simulink model "PWMGenerator"  (R2014b)
settings: Solver=ode45  StartTime=0.0  StopTime=2000  RelTol=1e-3
libraries: hdlsllib x15, simulink x5
settings Model: Creator=mchugh.ch  LastModifiedBy=sylvanus.a
settings OptimizationCC: UseDivisionForNetSlopeComputation=off  SimCompilerOptimization=off
settings DebuggingCC: FrameProcessingCompatibilityMsg=error
settings RTWCC: RTWCompilerOptimization=off
settings ConfigComp: CovMetricSettings=dw  CovHtmlReporting=on  CovSaveCumulativeToWorkspaceVar=on  CovSaveSingleToWorkspaceVar=on  CovModelRefEnable=Off  CovExternalEMLEnable=off  CovSFcnEnable=off

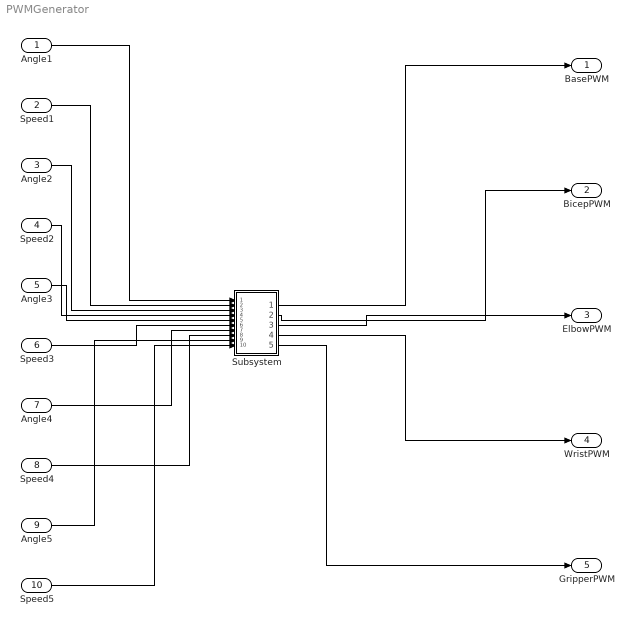
== system PWMGenerator ==
  Angle1 : Inport
  Speed1 : Inport  Port=2
  Angle2 : Inport  Port=3
  Speed2 : Inport  Port=4
  Angle3 : Inport  Port=5
  Speed3 : Inport  Port=6
  Angle4 : Inport  Port=7
  Speed4 : Inport  Port=8
  Angle5 : Inport  Port=9
  Speed5 : Inport  Port=10
  Subsystem : Subsystem  TreatAsAtomicUnit=on
  BasePWM : Outport  SampleTime=1
  BicepPWM : Outport  Port=2  SampleTime=1
  ElbowPWM : Outport  Port=3  SampleTime=1
  WristPWM : Outport  Port=4  SampleTime=1
  GripperPWM : Outport  Port=5  SampleTime=1
  wires:
  Angle1/1 -> Subsystem/1(Angle1)
  Speed1/1 -> Subsystem/2(Speed1)
  Angle2/1 -> Subsystem/3(Angle2)
  Speed2/1 -> Subsystem/4(Speed2)
  Angle3/1 -> Subsystem/5(Angle3)
  Speed3/1 -> Subsystem/6(Speed3)
  Angle4/1 -> Subsystem/7(Angle4)
  Speed4/1 -> Subsystem/8(Speed4)
  Angle5/1 -> Subsystem/9(Angle5)
  Speed5/1 -> Subsystem/10(Speed5)
  Subsystem/1(BasePWM) -> BasePWM/1
  Subsystem/2(BicepPWM) -> BicepPWM/1
  Subsystem/3(ElbowPWM) -> ElbowPWM/1
  Subsystem/4(WristPWM) -> WristPWM/1
  Subsystem/5(GripperPWM) -> GripperPWM/1

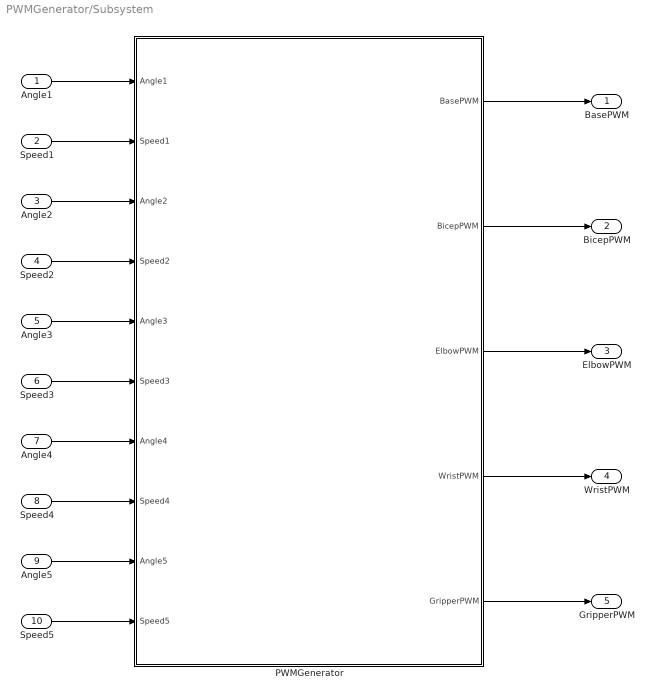
== system PWMGenerator/Subsystem ==
  Angle1 : Inport
  Speed1 : Inport  Port=2
  Angle2 : Inport  Port=3
  Speed2 : Inport  Port=4
  Angle3 : Inport  Port=5
  Speed3 : Inport  Port=6
  Angle4 : Inport  Port=7
  Speed4 : Inport  Port=8
  Angle5 : Inport  Port=9
  Speed5 : Inport  Port=10
  PWMGenerator : Subsystem
  BasePWM : Outport  SampleTime=1
  BicepPWM : Outport  Port=2  SampleTime=1
  ElbowPWM : Outport  Port=3  SampleTime=1
  WristPWM : Outport  Port=4  SampleTime=1
  GripperPWM : Outport  Port=5  SampleTime=1
  wires:
  Speed5/1 -> PWMGenerator/10(Speed5)
  PWMGenerator/5(GripperPWM) -> GripperPWM/1
  PWMGenerator/4(WristPWM) -> WristPWM/1
  PWMGenerator/2(BicepPWM) -> BicepPWM/1
  PWMGenerator/1(BasePWM) -> BasePWM/1
  PWMGenerator/3(ElbowPWM) -> ElbowPWM/1
  Speed3/1 -> PWMGenerator/6(Speed3)
  Angle3/1 -> PWMGenerator/5(Angle3)
  Angle2/1 -> PWMGenerator/3(Angle2)
  Speed1/1 -> PWMGenerator/2(Speed1)
  Angle4/1 -> PWMGenerator/7(Angle4)
  Speed4/1 -> PWMGenerator/8(Speed4)
  Angle5/1 -> PWMGenerator/9(Angle5)
  Angle1/1 -> PWMGenerator/1(Angle1)
  Speed2/1 -> PWMGenerator/4(Speed2)

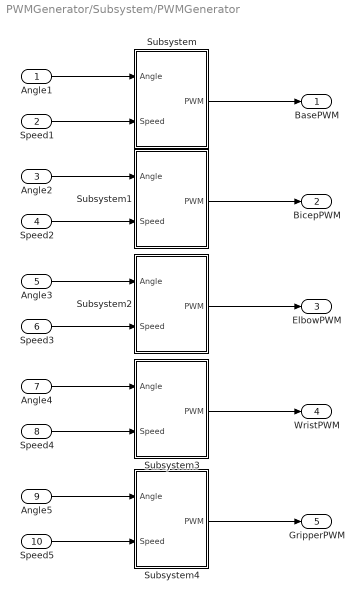
== system PWMGenerator/Subsystem/PWMGenerator ==
  Angle1 : Inport
  Speed1 : Inport  Port=2
  Angle2 : Inport  Port=3
  Speed2 : Inport  Port=4
  Angle3 : Inport  Port=5
  Speed3 : Inport  Port=6
  Angle4 : Inport  Port=7
  Speed4 : Inport  Port=8
  Angle5 : Inport  Port=9
  Speed5 : Inport  Port=10
  Subsystem : Subsystem  TreatAsAtomicUnit=on
  Subsystem1 : Subsystem  TreatAsAtomicUnit=on
  Subsystem2 : Subsystem  TreatAsAtomicUnit=on
  Subsystem3 : Subsystem  TreatAsAtomicUnit=on
  Subsystem4 : Subsystem  TreatAsAtomicUnit=on
  BasePWM : Outport  SampleTime=1
  BicepPWM : Outport  Port=2  SampleTime=1
  ElbowPWM : Outport  Port=3  SampleTime=1
  WristPWM : Outport  Port=4  SampleTime=1
  GripperPWM : Outport  Port=5  SampleTime=1
  wires:
  Speed1/1 -> Subsystem/2(Speed)
  Speed5/1 -> Subsystem4/2(Speed)
  Angle5/1 -> Subsystem4/1(Angle)
  Subsystem4/1(PWM) -> GripperPWM/1
  Angle1/1 -> Subsystem/1(Angle)
  Angle3/1 -> Subsystem2/1(Angle)
  Subsystem2/1(PWM) -> ElbowPWM/1
  Speed3/1 -> Subsystem2/2(Speed)
  Speed2/1 -> Subsystem1/2(Speed)
  Subsystem1/1(PWM) -> BicepPWM/1
  Angle2/1 -> Subsystem1/1(Angle)
  Subsystem3/1(PWM) -> WristPWM/1
  Angle4/1 -> Subsystem3/1(Angle)
  Speed4/1 -> Subsystem3/2(Speed)
  Subsystem/1(PWM) -> BasePWM/1

== system PWMGenerator/Subsystem/PWMGenerator/Subsystem ==
  Angle : Inport  OutDataTypeStr=uint32  SampleTime=1
  Speed : Inport  Port=2  OutDataTypeStr=uint32  SampleTime=1
  AngleSpeedToPWM : Subsystem
  Scope : Scope
  PWM : Outport  SampleTime=1
  wires:
  Speed/1 -> AngleSpeedToPWM/2(Speed)
  Angle/1 -> AngleSpeedToPWM/1(Angle)
  AngleSpeedToPWM/1(PWM) -> PWM/1, Scope/1

== system PWMGenerator/Subsystem/PWMGenerator/Subsystem1 ==
  Angle : Inport  OutDataTypeStr=uint32  SampleTime=1
  Speed : Inport  Port=2  OutDataTypeStr=uint32  SampleTime=1
  AngleSpeedToPWM : Subsystem
  Scope : Scope
  PWM : Outport  SampleTime=1
  wires:
  Speed/1 -> AngleSpeedToPWM/2(Speed)
  Angle/1 -> AngleSpeedToPWM/1(Angle)
  AngleSpeedToPWM/1(PWM) -> PWM/1, Scope/1

== system PWMGenerator/Subsystem/PWMGenerator/Subsystem2 ==
  Angle : Inport  OutDataTypeStr=uint32  SampleTime=1
  Speed : Inport  Port=2  OutDataTypeStr=uint32  SampleTime=1
  AngleSpeedToPWM : Subsystem
  Scope : Scope
  PWM : Outport  SampleTime=1
  wires:
  Speed/1 -> AngleSpeedToPWM/2(Speed)
  Angle/1 -> AngleSpeedToPWM/1(Angle)
  AngleSpeedToPWM/1(PWM) -> PWM/1, Scope/1

== system PWMGenerator/Subsystem/PWMGenerator/Subsystem3 ==
  Angle : Inport  OutDataTypeStr=uint32  SampleTime=1
  Speed : Inport  Port=2  OutDataTypeStr=uint32  SampleTime=1
  AngleSpeedToPWM : Subsystem
  Scope : Scope
  PWM : Outport  SampleTime=1
  wires:
  Speed/1 -> AngleSpeedToPWM/2(Speed)
  Angle/1 -> AngleSpeedToPWM/1(Angle)
  AngleSpeedToPWM/1(PWM) -> PWM/1, Scope/1

== system PWMGenerator/Subsystem/PWMGenerator/Subsystem4 ==
  Angle : Inport  OutDataTypeStr=uint32  SampleTime=1
  Speed : Inport  Port=2  OutDataTypeStr=uint32  SampleTime=1
  AngleSpeedToPWM : Subsystem
  Scope : Scope
  PWM : Outport  SampleTime=1
  wires:
  Speed/1 -> AngleSpeedToPWM/2(Speed)
  Angle/1 -> AngleSpeedToPWM/1(Angle)
  AngleSpeedToPWM/1(PWM) -> PWM/1, Scope/1

== system PWMGenerator/Subsystem/PWMGenerator/Subsystem/AngleSpeedToPWM ==
  Angle : Inport  OutDataTypeStr=uint32  SampleTime=1
  Speed : Inport  Port=2  OutDataTypeStr=uint32  SampleTime=1
  Subsystem : Subsystem
  PWM : Outport  SampleTime=1
  wires:
  Angle/1 -> Subsystem/1(Angle)
  Speed/1 -> Subsystem/2(Speed)
  Subsystem/1(PWM) -> PWM/1

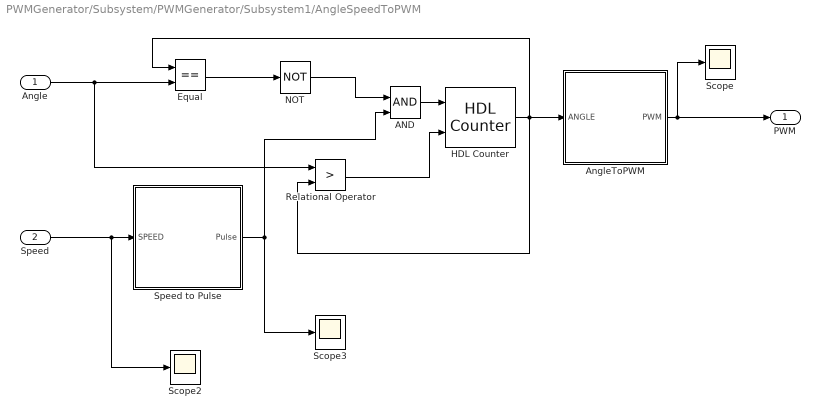
== system PWMGenerator/Subsystem/PWMGenerator/Subsystem1/AngleSpeedToPWM ==
  Angle : Inport  OutDataTypeStr=uint32  SampleTime=1
  Speed : Inport  Port=2  OutDataTypeStr=uint32  SampleTime=1
  AND : Logic  IconShape=distinctive  AllPortsSameDT=off  OutDataTypeStr=boolean
  AngleToPWM : Subsystem
  Equal : RelationalOperator  Operator===  OutDataTypeStr=boolean  SampleTime=1
  HDL Counter : hdlsllib/HDL Operations/HDL Counter  CountType=Count limited  CountInit=90  CountStep=1  CountMax=180  CountFromType=Specify  CountFrom=0  CountResetPort=off  CountLoadPort=off  CountEnbPort=on  CountDirPort=on  CountDataType=Unsigned  CountWordLen=32  CountFracLen=0  CountSampTime=1
  NOT : Logic  Operator=NOT  IconShape=distinctive  AllPortsSameDT=off  OutDataTypeStr=boolean
  Relational Operator : RelationalOperator  Operator=>  OutDataTypeStr=boolean
  Scope : Scope
      settings: SaveName=ScopeData5
  Scope2 : Scope
      settings: SaveName=ScopeData6
  Scope3 : Scope
      settings: SaveName=ScopeData7
  Speed to Pulse : Subsystem
  PWM : Outport  SampleTime=1
  wires:
  Equal/1 -> NOT/1
  HDL Counter/1 -> Relational Operator/2, Equal/1, AngleToPWM/1(ANGLE)
  AND/1 -> HDL Counter/1
  Speed/1 -> Scope2/1, Speed to Pulse/1(SPEED)
  Relational Operator/1 -> HDL Counter/2
  Speed to Pulse/1(Pulse) -> Scope3/1, AND/2
  NOT/1 -> AND/1
  AngleToPWM/1(PWM) -> PWM/1, Scope/1
  Angle/1 -> Equal/2, Relational Operator/1

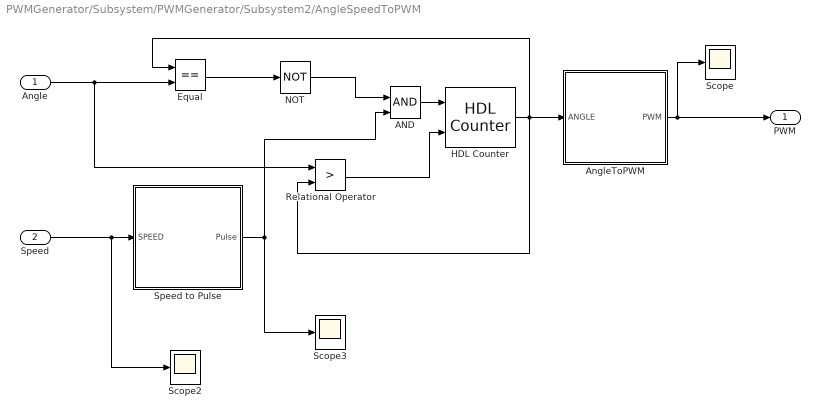
== system PWMGenerator/Subsystem/PWMGenerator/Subsystem2/AngleSpeedToPWM ==
  Angle : Inport  OutDataTypeStr=uint32  SampleTime=1
  Speed : Inport  Port=2  OutDataTypeStr=uint32  SampleTime=1
  AND : Logic  IconShape=distinctive  AllPortsSameDT=off  OutDataTypeStr=boolean
  AngleToPWM : Subsystem
  Equal : RelationalOperator  Operator===  OutDataTypeStr=boolean  SampleTime=1
  HDL Counter : hdlsllib/HDL Operations/HDL Counter  CountType=Count limited  CountInit=90  CountStep=1  CountMax=180  CountFromType=Specify  CountFrom=0  CountResetPort=off  CountLoadPort=off  CountEnbPort=on  CountDirPort=on  CountDataType=Unsigned  CountWordLen=32  CountFracLen=0  CountSampTime=1
  NOT : Logic  Operator=NOT  IconShape=distinctive  AllPortsSameDT=off  OutDataTypeStr=boolean
  Relational Operator : RelationalOperator  Operator=>  OutDataTypeStr=boolean
  Scope : Scope
      settings: SaveName=ScopeData5
  Scope2 : Scope
      settings: SaveName=ScopeData6
  Scope3 : Scope
      settings: SaveName=ScopeData7
  Speed to Pulse : Subsystem
  PWM : Outport  SampleTime=1
  wires:
  Equal/1 -> NOT/1
  HDL Counter/1 -> Relational Operator/2, Equal/1, AngleToPWM/1(ANGLE)
  AND/1 -> HDL Counter/1
  Speed/1 -> Scope2/1, Speed to Pulse/1(SPEED)
  Relational Operator/1 -> HDL Counter/2
  Speed to Pulse/1(Pulse) -> Scope3/1, AND/2
  NOT/1 -> AND/1
  AngleToPWM/1(PWM) -> PWM/1, Scope/1
  Angle/1 -> Equal/2, Relational Operator/1

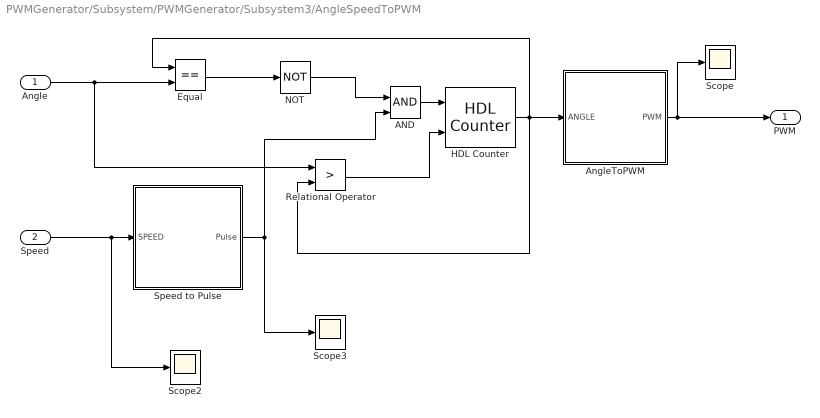
== system PWMGenerator/Subsystem/PWMGenerator/Subsystem3/AngleSpeedToPWM ==
  Angle : Inport  OutDataTypeStr=uint32  SampleTime=1
  Speed : Inport  Port=2  OutDataTypeStr=uint32  SampleTime=1
  AND : Logic  IconShape=distinctive  AllPortsSameDT=off  OutDataTypeStr=boolean
  AngleToPWM : Subsystem
  Equal : RelationalOperator  Operator===  OutDataTypeStr=boolean  SampleTime=1
  HDL Counter : hdlsllib/HDL Operations/HDL Counter  CountType=Count limited  CountInit=90  CountStep=1  CountMax=180  CountFromType=Specify  CountFrom=0  CountResetPort=off  CountLoadPort=off  CountEnbPort=on  CountDirPort=on  CountDataType=Unsigned  CountWordLen=32  CountFracLen=0  CountSampTime=1
  NOT : Logic  Operator=NOT  IconShape=distinctive  AllPortsSameDT=off  OutDataTypeStr=boolean
  Relational Operator : RelationalOperator  Operator=>  OutDataTypeStr=boolean
  Scope : Scope
      settings: SaveName=ScopeData5
  Scope2 : Scope
      settings: SaveName=ScopeData6
  Scope3 : Scope
      settings: SaveName=ScopeData7
  Speed to Pulse : Subsystem
  PWM : Outport  SampleTime=1
  wires:
  Equal/1 -> NOT/1
  HDL Counter/1 -> Relational Operator/2, Equal/1, AngleToPWM/1(ANGLE)
  AND/1 -> HDL Counter/1
  Speed/1 -> Scope2/1, Speed to Pulse/1(SPEED)
  Relational Operator/1 -> HDL Counter/2
  Speed to Pulse/1(Pulse) -> Scope3/1, AND/2
  NOT/1 -> AND/1
  AngleToPWM/1(PWM) -> PWM/1, Scope/1
  Angle/1 -> Equal/2, Relational Operator/1

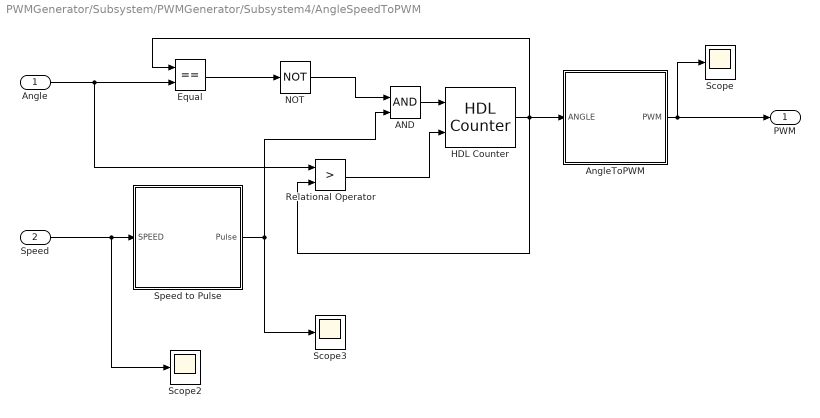
== system PWMGenerator/Subsystem/PWMGenerator/Subsystem4/AngleSpeedToPWM ==
  Angle : Inport  OutDataTypeStr=uint32  SampleTime=1
  Speed : Inport  Port=2  OutDataTypeStr=uint32  SampleTime=1
  AND : Logic  IconShape=distinctive  AllPortsSameDT=off  OutDataTypeStr=boolean
  AngleToPWM : Subsystem
  Equal : RelationalOperator  Operator===  OutDataTypeStr=boolean  SampleTime=1
  HDL Counter : hdlsllib/HDL Operations/HDL Counter  CountType=Count limited  CountInit=90  CountStep=1  CountMax=180  CountFromType=Specify  CountFrom=0  CountResetPort=off  CountLoadPort=off  CountEnbPort=on  CountDirPort=on  CountDataType=Unsigned  CountWordLen=32  CountFracLen=0  CountSampTime=1
  NOT : Logic  Operator=NOT  IconShape=distinctive  AllPortsSameDT=off  OutDataTypeStr=boolean
  Relational Operator : RelationalOperator  Operator=>  OutDataTypeStr=boolean
  Scope : Scope
      settings: SaveName=ScopeData5
  Scope2 : Scope
      settings: SaveName=ScopeData6
  Scope3 : Scope
      settings: SaveName=ScopeData7
  Speed to Pulse : Subsystem
  PWM : Outport  SampleTime=1
  wires:
  Equal/1 -> NOT/1
  HDL Counter/1 -> Relational Operator/2, Equal/1, AngleToPWM/1(ANGLE)
  AND/1 -> HDL Counter/1
  Speed/1 -> Scope2/1, Speed to Pulse/1(SPEED)
  Relational Operator/1 -> HDL Counter/2
  Speed to Pulse/1(Pulse) -> Scope3/1, AND/2
  NOT/1 -> AND/1
  AngleToPWM/1(PWM) -> PWM/1, Scope/1
  Angle/1 -> Equal/2, Relational Operator/1

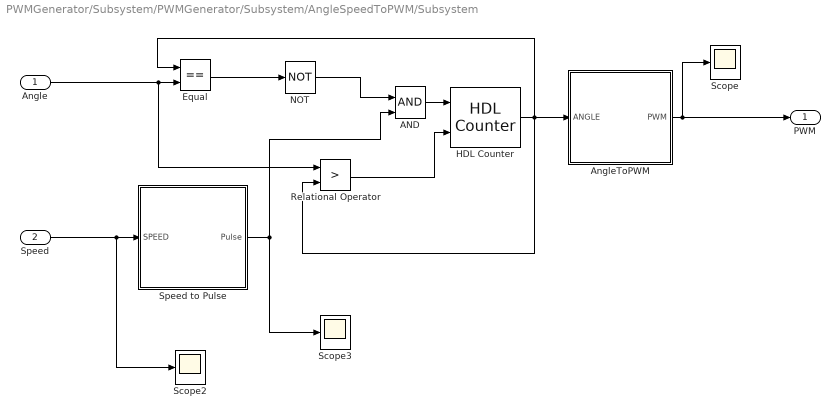
== system PWMGenerator/Subsystem/PWMGenerator/Subsystem/AngleSpeedToPWM/Subsystem ==
  Angle : Inport  OutDataTypeStr=uint32  SampleTime=1
  Speed : Inport  Port=2  OutDataTypeStr=uint32  SampleTime=1
  AND : Logic  IconShape=distinctive  AllPortsSameDT=off  OutDataTypeStr=boolean
  AngleToPWM : Subsystem
  Equal : RelationalOperator  Operator===  OutDataTypeStr=boolean  SampleTime=1
  HDL Counter : hdlsllib/HDL Operations/HDL Counter  CountType=Count limited  CountInit=90  CountStep=1  CountMax=180  CountFromType=Specify  CountFrom=0  CountResetPort=off  CountLoadPort=off  CountEnbPort=on  CountDirPort=on  CountDataType=Unsigned  CountWordLen=32  CountFracLen=0  CountSampTime=1
  NOT : Logic  Operator=NOT  IconShape=distinctive  AllPortsSameDT=off  OutDataTypeStr=boolean
  Relational Operator : RelationalOperator  Operator=>  OutDataTypeStr=boolean
  Scope : Scope
      settings: SaveName=ScopeData5
  Scope2 : Scope
      settings: SaveName=ScopeData6
  Scope3 : Scope
      settings: SaveName=ScopeData7
  Speed to Pulse : Subsystem
  PWM : Outport  SampleTime=1
  wires:
  Equal/1 -> NOT/1
  HDL Counter/1 -> Relational Operator/2, Equal/1, AngleToPWM/1(ANGLE)
  AND/1 -> HDL Counter/1
  Speed/1 -> Scope2/1, Speed to Pulse/1(SPEED)
  Relational Operator/1 -> HDL Counter/2
  Speed to Pulse/1(Pulse) -> Scope3/1, AND/2
  NOT/1 -> AND/1
  AngleToPWM/1(PWM) -> PWM/1, Scope/1
  Angle/1 -> Relational Operator/1, Equal/2

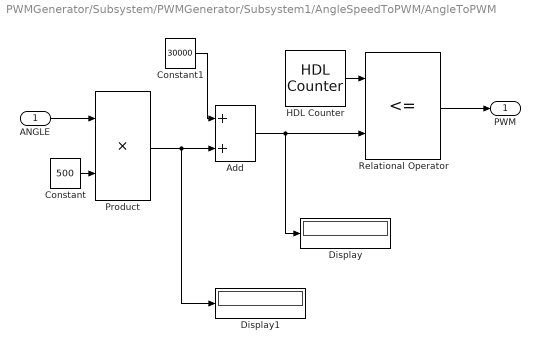
== system PWMGenerator/Subsystem/PWMGenerator/Subsystem1/AngleSpeedToPWM/AngleToPWM ==
  ANGLE : Inport  OutDataTypeStr=uint32
  Add : Sum  OutDataTypeStr=uint32
  Constant : Constant  Value=500  OutDataTypeStr=uint32
  Constant1 : Constant  Value=30000  OutDataTypeStr=uint32
  Display : Display
  Display1 : Display
  HDL Counter : hdlsllib/HDL Operations/HDL Counter  CountType=Count limited  CountInit=0  CountStep=1  CountMax=1000000  CountFromType=Initial value  CountFrom=0  CountResetPort=off  CountLoadPort=off  CountEnbPort=off  CountDirPort=off  CountDataType=Unsigned  CountWordLen=32  CountFracLen=0  CountSampTime=1
  Product : Product  OutDataTypeStr=uint32  SaturateOnIntegerOverflow=on  RndMeth=Zero
  Relational Operator : RelationalOperator  Operator=<=  OutDataTypeStr=boolean  SampleTime=1
  PWM : Outport  SampleTime=1
  wires:
  HDL Counter/1 -> Relational Operator/1
  Product/1 -> Display1/1, Add/2
  ANGLE/1 -> Product/1
  Constant/1 -> Product/2
  Constant1/1 -> Add/1
  Add/1 -> Display/1, Relational Operator/2
  Relational Operator/1 -> PWM/1

== system PWMGenerator/Subsystem/PWMGenerator/Subsystem1/AngleSpeedToPWM/Speed to Pulse ==
  SPEED : Inport  OutDataTypeStr=uint32  SampleTime=1
  Compare To Constant : simulink/Logic and Bit Operations/Compare To Constant  relop===  const=0  OutDataTypeStr=boolean
  Constant : Constant  Value=50000000  OutDataTypeStr=uint32
  Display : Display
  Divide : Product  Inputs=*/  OutDataTypeStr=uint32  SaturateOnIntegerOverflow=on  RndMeth=Zero
  HDL Counter : hdlsllib/HDL Operations/HDL Counter  CountType=Count limited  CountInit=0  CountStep=1  CountMax=50000000  CountFromType=Initial value  CountFrom=0  CountResetPort=on  CountLoadPort=off  CountEnbPort=off  CountDirPort=off  CountDataType=Unsigned  CountWordLen=32  CountFracLen=0  CountSampTime=1
  Relational Operator : RelationalOperator  OutDataTypeStr=boolean
  Scope : Scope
      settings: TimeRange=2000
  Pulse : Outport  OutDataTypeStr=boolean
  wires:
  Compare To Constant/1 -> Scope/1, Pulse/1
  HDL Counter/1 -> Relational Operator/1, Compare To Constant/1
  Constant/1 -> Divide/1
  Divide/1 -> Relational Operator/2, Display/1
  Relational Operator/1 -> HDL Counter/1
  SPEED/1 -> Divide/2

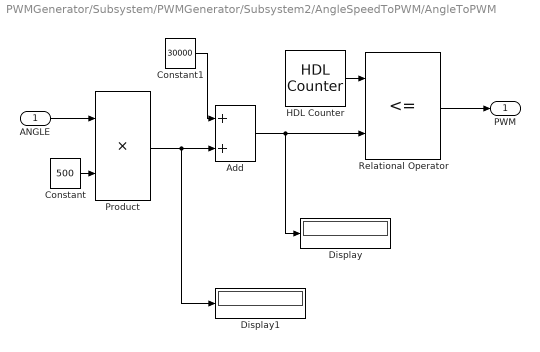
== system PWMGenerator/Subsystem/PWMGenerator/Subsystem2/AngleSpeedToPWM/AngleToPWM ==
  ANGLE : Inport  OutDataTypeStr=uint32
  Add : Sum  OutDataTypeStr=uint32
  Constant : Constant  Value=500  OutDataTypeStr=uint32
  Constant1 : Constant  Value=30000  OutDataTypeStr=uint32
  Display : Display
  Display1 : Display
  HDL Counter : hdlsllib/HDL Operations/HDL Counter  CountType=Count limited  CountInit=0  CountStep=1  CountMax=1000000  CountFromType=Initial value  CountFrom=0  CountResetPort=off  CountLoadPort=off  CountEnbPort=off  CountDirPort=off  CountDataType=Unsigned  CountWordLen=32  CountFracLen=0  CountSampTime=1
  Product : Product  OutDataTypeStr=uint32  SaturateOnIntegerOverflow=on  RndMeth=Zero
  Relational Operator : RelationalOperator  Operator=<=  OutDataTypeStr=boolean  SampleTime=1
  PWM : Outport  SampleTime=1
  wires:
  HDL Counter/1 -> Relational Operator/1
  Product/1 -> Display1/1, Add/2
  ANGLE/1 -> Product/1
  Constant/1 -> Product/2
  Constant1/1 -> Add/1
  Add/1 -> Display/1, Relational Operator/2
  Relational Operator/1 -> PWM/1

== system PWMGenerator/Subsystem/PWMGenerator/Subsystem2/AngleSpeedToPWM/Speed to Pulse ==
  SPEED : Inport  OutDataTypeStr=uint32  SampleTime=1
  Compare To Constant : simulink/Logic and Bit Operations/Compare To Constant  relop===  const=0  OutDataTypeStr=boolean
  Constant : Constant  Value=50000000  OutDataTypeStr=uint32
  Display : Display
  Divide : Product  Inputs=*/  OutDataTypeStr=uint32  SaturateOnIntegerOverflow=on  RndMeth=Zero
  HDL Counter : hdlsllib/HDL Operations/HDL Counter  CountType=Count limited  CountInit=0  CountStep=1  CountMax=50000000  CountFromType=Initial value  CountFrom=0  CountResetPort=on  CountLoadPort=off  CountEnbPort=off  CountDirPort=off  CountDataType=Unsigned  CountWordLen=32  CountFracLen=0  CountSampTime=1
  Relational Operator : RelationalOperator  OutDataTypeStr=boolean
  Scope : Scope
      settings: TimeRange=2000
  Pulse : Outport  OutDataTypeStr=boolean
  wires:
  Compare To Constant/1 -> Scope/1, Pulse/1
  HDL Counter/1 -> Relational Operator/1, Compare To Constant/1
  Constant/1 -> Divide/1
  Divide/1 -> Relational Operator/2, Display/1
  Relational Operator/1 -> HDL Counter/1
  SPEED/1 -> Divide/2

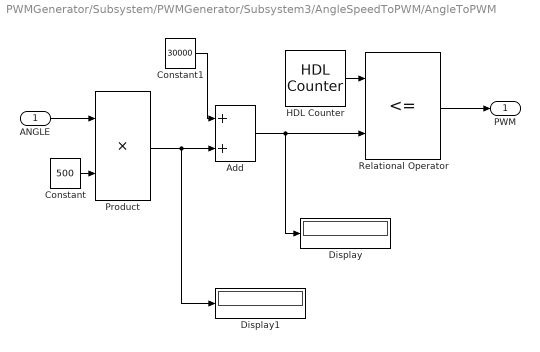
== system PWMGenerator/Subsystem/PWMGenerator/Subsystem3/AngleSpeedToPWM/AngleToPWM ==
  ANGLE : Inport  OutDataTypeStr=uint32
  Add : Sum  OutDataTypeStr=uint32
  Constant : Constant  Value=500  OutDataTypeStr=uint32
  Constant1 : Constant  Value=30000  OutDataTypeStr=uint32
  Display : Display
  Display1 : Display
  HDL Counter : hdlsllib/HDL Operations/HDL Counter  CountType=Count limited  CountInit=0  CountStep=1  CountMax=1000000  CountFromType=Initial value  CountFrom=0  CountResetPort=off  CountLoadPort=off  CountEnbPort=off  CountDirPort=off  CountDataType=Unsigned  CountWordLen=32  CountFracLen=0  CountSampTime=1
  Product : Product  OutDataTypeStr=uint32  SaturateOnIntegerOverflow=on  RndMeth=Zero
  Relational Operator : RelationalOperator  Operator=<=  OutDataTypeStr=boolean  SampleTime=1
  PWM : Outport  SampleTime=1
  wires:
  HDL Counter/1 -> Relational Operator/1
  Product/1 -> Display1/1, Add/2
  ANGLE/1 -> Product/1
  Constant/1 -> Product/2
  Constant1/1 -> Add/1
  Add/1 -> Display/1, Relational Operator/2
  Relational Operator/1 -> PWM/1

== system PWMGenerator/Subsystem/PWMGenerator/Subsystem3/AngleSpeedToPWM/Speed to Pulse ==
  SPEED : Inport  OutDataTypeStr=uint32  SampleTime=1
  Compare To Constant : simulink/Logic and Bit Operations/Compare To Constant  relop===  const=0  OutDataTypeStr=boolean
  Constant : Constant  Value=50000000  OutDataTypeStr=uint32
  Display : Display
  Divide : Product  Inputs=*/  OutDataTypeStr=uint32  SaturateOnIntegerOverflow=on  RndMeth=Zero
  HDL Counter : hdlsllib/HDL Operations/HDL Counter  CountType=Count limited  CountInit=0  CountStep=1  CountMax=50000000  CountFromType=Initial value  CountFrom=0  CountResetPort=on  CountLoadPort=off  CountEnbPort=off  CountDirPort=off  CountDataType=Unsigned  CountWordLen=32  CountFracLen=0  CountSampTime=1
  Relational Operator : RelationalOperator  OutDataTypeStr=boolean
  Scope : Scope
      settings: TimeRange=2000
  Pulse : Outport  OutDataTypeStr=boolean
  wires:
  Compare To Constant/1 -> Scope/1, Pulse/1
  HDL Counter/1 -> Relational Operator/1, Compare To Constant/1
  Constant/1 -> Divide/1
  Divide/1 -> Relational Operator/2, Display/1
  Relational Operator/1 -> HDL Counter/1
  SPEED/1 -> Divide/2

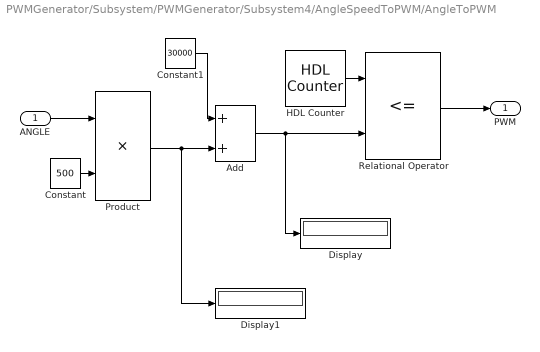
== system PWMGenerator/Subsystem/PWMGenerator/Subsystem4/AngleSpeedToPWM/AngleToPWM ==
  ANGLE : Inport  OutDataTypeStr=uint32
  Add : Sum  OutDataTypeStr=uint32
  Constant : Constant  Value=500  OutDataTypeStr=uint32
  Constant1 : Constant  Value=30000  OutDataTypeStr=uint32
  Display : Display
  Display1 : Display
  HDL Counter : hdlsllib/HDL Operations/HDL Counter  CountType=Count limited  CountInit=0  CountStep=1  CountMax=1000000  CountFromType=Initial value  CountFrom=0  CountResetPort=off  CountLoadPort=off  CountEnbPort=off  CountDirPort=off  CountDataType=Unsigned  CountWordLen=32  CountFracLen=0  CountSampTime=1
  Product : Product  OutDataTypeStr=uint32  SaturateOnIntegerOverflow=on  RndMeth=Zero
  Relational Operator : RelationalOperator  Operator=<=  OutDataTypeStr=boolean  SampleTime=1
  PWM : Outport  SampleTime=1
  wires:
  HDL Counter/1 -> Relational Operator/1
  Product/1 -> Display1/1, Add/2
  ANGLE/1 -> Product/1
  Constant/1 -> Product/2
  Constant1/1 -> Add/1
  Add/1 -> Display/1, Relational Operator/2
  Relational Operator/1 -> PWM/1

== system PWMGenerator/Subsystem/PWMGenerator/Subsystem4/AngleSpeedToPWM/Speed to Pulse ==
  SPEED : Inport  OutDataTypeStr=uint32  SampleTime=1
  Compare To Constant : simulink/Logic and Bit Operations/Compare To Constant  relop===  const=0  OutDataTypeStr=boolean
  Constant : Constant  Value=50000000  OutDataTypeStr=uint32
  Display : Display
  Divide : Product  Inputs=*/  OutDataTypeStr=uint32  SaturateOnIntegerOverflow=on  RndMeth=Zero
  HDL Counter : hdlsllib/HDL Operations/HDL Counter  CountType=Count limited  CountInit=0  CountStep=1  CountMax=50000000  CountFromType=Initial value  CountFrom=0  CountResetPort=on  CountLoadPort=off  CountEnbPort=off  CountDirPort=off  CountDataType=Unsigned  CountWordLen=32  CountFracLen=0  CountSampTime=1
  Relational Operator : RelationalOperator  OutDataTypeStr=boolean
  Scope : Scope
      settings: TimeRange=2000
  Pulse : Outport  OutDataTypeStr=boolean
  wires:
  Compare To Constant/1 -> Scope/1, Pulse/1
  HDL Counter/1 -> Relational Operator/1, Compare To Constant/1
  Constant/1 -> Divide/1
  Divide/1 -> Relational Operator/2, Display/1
  Relational Operator/1 -> HDL Counter/1
  SPEED/1 -> Divide/2

== system PWMGenerator/Subsystem/PWMGenerator/Subsystem/AngleSpeedToPWM/Subsystem/AngleToPWM ==
  ANGLE : Inport  OutDataTypeStr=uint32
  Add : Sum  OutDataTypeStr=uint32
  Constant : Constant  Value=500  OutDataTypeStr=uint32
  Constant1 : Constant  Value=30000  OutDataTypeStr=uint32
  Display : Display
  Display1 : Display
  HDL Counter : hdlsllib/HDL Operations/HDL Counter  CountType=Count limited  CountInit=0  CountStep=1  CountMax=1000000  CountFromType=Initial value  CountFrom=0  CountResetPort=off  CountLoadPort=off  CountEnbPort=off  CountDirPort=off  CountDataType=Unsigned  CountWordLen=32  CountFracLen=0  CountSampTime=1
  Product : Product  OutDataTypeStr=uint32  SaturateOnIntegerOverflow=on  RndMeth=Zero
  Relational Operator : RelationalOperator  Operator=<=  OutDataTypeStr=boolean  SampleTime=1
  PWM : Outport  SampleTime=1
  wires:
  HDL Counter/1 -> Relational Operator/1
  Product/1 -> Display1/1, Add/2
  ANGLE/1 -> Product/1
  Constant/1 -> Product/2
  Constant1/1 -> Add/1
  Add/1 -> Display/1, Relational Operator/2
  Relational Operator/1 -> PWM/1

== system PWMGenerator/Subsystem/PWMGenerator/Subsystem/AngleSpeedToPWM/Subsystem/Speed to Pulse ==
  SPEED : Inport  OutDataTypeStr=uint32  SampleTime=1
  Compare To Constant : simulink/Logic and Bit Operations/Compare To Constant  relop===  const=0  OutDataTypeStr=boolean
  Constant : Constant  Value=50000000  OutDataTypeStr=uint32
  Display : Display
  Divide : Product  Inputs=*/  SaturateOnIntegerOverflow=on  RndMeth=Zero
  HDL Counter : hdlsllib/HDL Operations/HDL Counter  CountType=Count limited  CountInit=0  CountStep=1  CountMax=50000000  CountFromType=Initial value  CountFrom=0  CountResetPort=on  CountLoadPort=off  CountEnbPort=off  CountDirPort=off  CountDataType=Unsigned  CountWordLen=32  CountFracLen=0  CountSampTime=1
  Relational Operator : RelationalOperator  OutDataTypeStr=boolean
  Scope : Scope
      settings: TimeRange=2000
  Pulse : Outport  OutDataTypeStr=boolean
  wires:
  Compare To Constant/1 -> Scope/1, Pulse/1
  HDL Counter/1 -> Relational Operator/1, Compare To Constant/1
  Constant/1 -> Divide/1
  Divide/1 -> Relational Operator/2, Display/1
  Relational Operator/1 -> HDL Counter/1
  SPEED/1 -> Divide/2
